simulink model "model_sim2014"  (R2014a)
settings: Solver=ode4  StartTime=0.0  StopTime=40  FixedStep=0.01  RelTol=1e-3
values from neighbouring files (symbols this model uses):
  K = X0(1)    [cel.m]    (also in cel_t.m; lsm.m = par(1); lsm_tarcie.m = par(1))
  T = X0(2)    [cel.m]    (also in cel_t.m; lsm.m = par(2); lsm_tarcie.m = par(2))
  tau = X0(3)    [cel.m]    (also in cel_t.m; lsm.m = par(3); lsm_tarcie.m = par(3))
settings Model: CovModelRefEnable=off  CovSFcnEnable=on  Creator=Maciek  LastModifiedBy=Maciek
settings DataIOCC: LimitDataPoints=off  SaveFormat=StructureWithTime
settings DebuggingCC: MergeDetectMultiDrivingBlocksExec=error  SolverPrmCheckMsg=none  FrameProcessingCompatibilityMsg=error
settings HardwareCC: ProdBitPerPointer=64  ProdLargestAtomicFloat=Float  ProdIntDivRoundTo=Zero  ProdEndianess=LittleEndian  ProdHWDeviceType=Specified
settings ModelReferenceCC: PropagateSignalLabelsOutOfModel=on

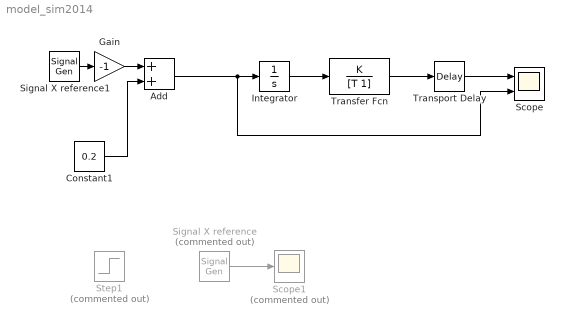
== system model_sim2014 ==
  Add : Sum
  Constant1 : Constant  Value=0.2
  Gain : Gain  Gain=-1
  Integrator : Integrator
  Scope : Scope  NumInputPorts=2
      settings: TimeRange=auto  MaxDataPoints=5000  SaveName=data  YMin=-0.05382~-0.026  YMax=0.48437~0.234  SampleTime=-1
  Scope1 : Scope  Commented=on
      settings: TimeRange=auto  MaxDataPoints=5000  SaveToWorkspace=off  YMin=-0.02499  YMax=0.025  SampleTime=-1
  Signal X reference : SignalGenerator  Commented=on  WaveForm=sawtooth  Amplitude=0.02  Frequency=0.06
  Signal X reference1 : SignalGenerator  WaveForm=sawtooth  Amplitude=0.2  Frequency=0.02
  Step1 : Step  Commented=on  Time=20  After=-1  SampleTime=0
  Transfer Fcn : TransferFcn  Numerator=K  Denominator=[T 1]
  Transport Delay : TransportDelay  DelayTime=tau
  wires:
  Integrator/1 -> Transfer Fcn/1
  Constant1/1 -> Add/2
  Signal X reference/1 -> Scope1/1
  Transfer Fcn/1 -> Transport Delay/1
  Add/1 -> Scope/2, Integrator/1
  Signal X reference1/1 -> Gain/1
  Gain/1 -> Add/1
  Transport Delay/1 -> Scope/1
